simulink model "LookupTableWithFakeValues"  (R2024b)
settings: Solver=VariableStepAuto  StartTime=0.0  StopTime=10.0  RelTol=1e-3
undefined symbols (not defined in the file): Q_targets, RPM1_grid, RPM2_grid, T_targets
settings Model: Creator=alyssasanden  LastModifiedBy=alyssasanden

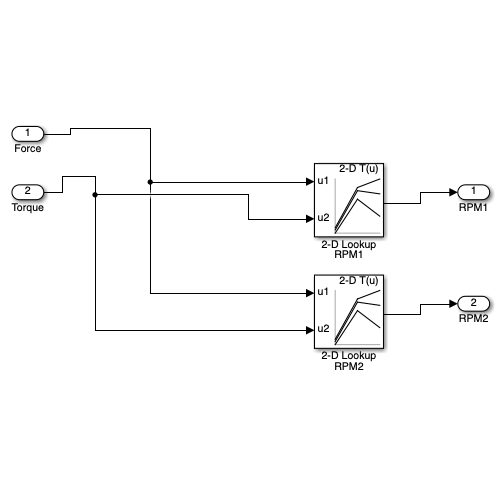
[thumbnail: Simulink's stored preview of the top-level diagram]
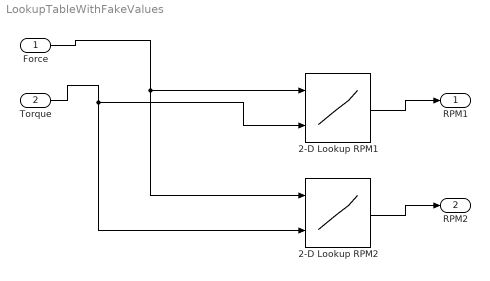
== system LookupTableWithFakeValues ==
  Force : Inport
  Torque : Inport  Port=2
  2-D Lookup RPM1 : Lookup_n-D  BreakpointsForDimension1=T_targets  BreakpointsForDimension2=Q_targets  Table=RPM1_grid  InternalRulePriority=Speed  RndMeth=Simplest
      settings: InputPortMap=u0,u1
  2-D Lookup RPM2 : Lookup_n-D  BreakpointsForDimension1=T_targets  BreakpointsForDimension2=Q_targets  Table=RPM2_grid  InternalRulePriority=Speed  RndMeth=Simplest
      settings: InputPortMap=u0,u1
  RPM1 : Outport
  RPM2 : Outport  Port=2
  wires:
  2-D Lookup RPM1/1 -> RPM1/1
  2-D Lookup RPM2/1 -> RPM2/1
  Force/1 -> 2-D Lookup RPM2/1, 2-D Lookup RPM1/1
  Torque/1 -> 2-D Lookup RPM2/2, 2-D Lookup RPM1/2
